simulink model "PFC_69C_03_06_V01_3Phase_3_2KW"  (R2022b)
settings: Solver=FixedStepAuto  StartTime=0.0  StopTime=Inf  RelTol=1e-3  EnableMultiTasking=on
model workspace (MAT data in the model file):
  ADC_Gain = 1241.21212121
  DAC_Gain = 0.000805860805861
  Inductor_Current_Divider_Gain_Phase_A = 33.4
  Inductor_Current_Divider_Gain_Phase_B = 33.4
  Vbulk_Divider_Gain = 276.854928018
  Vin_Divider_Gain = 556.17352614
undefined symbols (not defined in the file or in its folder): GPTRIP1SEL, GPTRIP2SEL, SCI_A_Transmit, SCI_A_Transmit_Current_Suffix, SCI_A_Transmit_one_shot_Suffix, SCI_A_Transmit_Polarity_Suffix, SCI_A_Transmit_relay_Suffix, SCI_A_Transmit_Vbulk_Suffix, SCI_A_Transmit_Vin_rms_Suffix, SCI_A_Transmit_Vin_Suffix, SCI_A_Transmit_Vmid_Suffix, SCI_A_Transmit_Vp_Suffix, SCI_A_Transmit_Vpfc_Suffix, TZ1, TZ2
libraries: c280xlib x38, c2802xlib x34, simulink x17, c2000lib x1
(part 8 of 8)

== stateflow chart PFC_69C_03_06_V01_3Phase_3_2KW/Calibration,RMS, Fault Protection @5kHz/Fault checking/If Action Subsystem/PFC_en_update_Phase_B/Chart ==
  note: Local variables
      | VbusRefTemp
      | SoftStartCnt
  note: Verror = Vbulk_Ref_ADC_adjusted - Vbulk_ADC;
  (default) -> (junction 47)
  (junction 47) -> (junction 50) [order 4]
  (junction 47) -> (junction 68) [order 1] : [Vin_OVP_Flag]
  (junction 68) -> (junction 80) : {PFC_en=0;}
  (junction 47) -> (junction 15) [order 2] : [Iin_OCP_Flag]
  (junction 50) -> (junction 52) : {
      | PFC_en=1;
      | PFC_en1=1;
      | }
  (junction 47) -> (junction 5) [order 3] : [Vin_UVP_Flag]
  (junction 80) -> (junction 82)
  (junction 82) -> (junction 84)
  (junction 5) -> (junction 38) : {
      | PFC_en=0;
      | PFC_en1=0;
      | }
  (junction 15) -> (junction 20) : {PFC_en=0;
      | PFC_en1=0;}
  (junction 52) -> (junction 38)
  (junction 20) -> (junction 38)
  (junction 84) -> (junction 20)
  data: Vin_UVP_Flag input; VbusRefTemp local =0; Vin_OVP_Flag input; SoftStartCnt local =0; Vbulk_Ref_ADC_Hard_Value local =0; UVPCnt local =0; PFC_en output; PFC_en1 output; Iin_OCP_Flag input; Iin_OCP_Flag1 local
